simulink model "verify_Ventilation_AIV_mdl"  (R2016b)
settings: Solver=VariableStepDiscrete  StartTime=0  StopTime=1  MaxStep=1  RelTol=1e-3  EnableMultiTasking=on
undefined symbols (not defined in the file or in its folder): density, heat_capacity, rel_hum2x
libraries: carnot x3
settings Model: Creator=drhf  LastModifiedBy=drhf
settings DataIOCC: SaveFormat=Array  SignalLoggingSaveFormat=ModelDataLogs
settings OptimizationCC: ExpressionDepthLimit=2147483647  LifeSpan=inf
settings DebuggingCC: UnderspecifiedInitializationDetection=Classic  MergeDetectMultiDrivingBlocksExec=none  SolverPrmCheckMsg=warning  FcnCallInpInsideContextMsg=warning  StateNameClashWarn=warning  SFUnexpectedBacktrackingDiag=warning  SFNoUnconditionalDefaultTransitionDiag=warning  SFExecutionAtInitializationDiag=none
settings HardwareCC: ProdBitPerPointer=32  ProdBitPerSizeT=32  ProdBitPerPtrDiffT=32  ProdLargestAtomicFloat=None  ProdIntDivRoundTo=Undefined  ProdEndianess=Unspecified  ProdWordSize=32  ProdHWDeviceType=32-bit Generic
settings ModelReferenceCC: PropagateSignalLabelsOutOfModel=off
settings GRTTargetCC: TargetLangStandard=C89/C90 (ANSI)  GeneratePreprocessorConditionals=Disable all  CombineOutputUpdateFcns=off  GRTInterface=on
settings ConfigComp: CovMetricSettings=dw  CovHtmlReporting=on  CovSaveCumulativeToWorkspaceVar=on  CovSaveSingleToWorkspaceVar=on  CovExternalEMLEnable=off

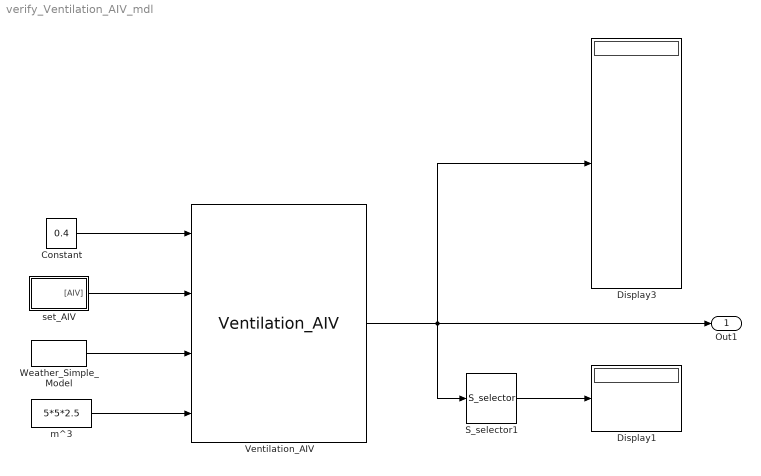
== system verify_Ventilation_AIV_mdl ==
  Constant : Constant  Value=0.4
  Display1 : Display
  Display3 : Display
  S_selector1 : carnot/Outputs/S_selector  e1=off  e2=off  e3=off  e4=off  e5=off  e6=off  e7=off  e8=off  e9=on  e10=on  e11=on  e12=off  e13=off
  Ventilation_AIV : carnot/Source/Ventilation/Ventilation_AIV  co2=400
  Weather_Simple_Model : carnot/Weather/Weather_Simple_Model  lat=60  Ibn=900  Idg=100  tamb=0  deltaTsky=0  rh=50  precip="10e-3/24/3600           % 10 mm in 24 h"  cloud=0.125  p=1013e2  vw=1  wdir=270
  m^3 : Constant  Value=5*5*2.5
  set_AIV : Subsystem
  Out1 : Outport
  wires:
  Constant/1 -> Ventilation_AIV/1
  set_AIV/1("[AIV]") -> Ventilation_AIV/2
  Weather_Simple_Model/1 -> Ventilation_AIV/3
  Ventilation_AIV/1 -> S_selector1/1, Display3/1, Out1/1
  m^3/1 -> Ventilation_AIV/4
  S_selector1/1 -> Display1/1

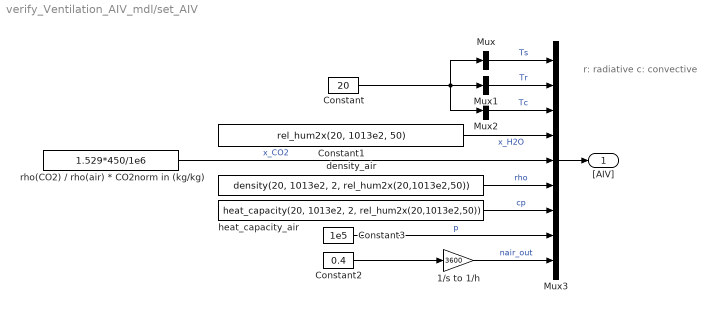
== system verify_Ventilation_AIV_mdl/set_AIV ==
  note: r: radiative
      | c: convective
  1/s to 1/h : Gain  Gain=3600  SaturateOnIntegerOverflow=on  OutDataTypeStr=Inherit: Same as input  ParamDataTypeStr=Inherit: Same as input
  Constant : Constant  Value=20
  Constant1 : Constant  Value=rel_hum2x(20, 1013e2, 50)
  Constant2 : Constant  Value=0.4
  Constant3 : Constant  Value=1e5
  Mux : Mux  Inputs=1
  Mux1 : Mux  Inputs=1
  Mux2 : Mux  Inputs=1
  Mux3 : Mux  Inputs=9
  density_air : Constant  Value=density(20, 1013e2, 2, rel_hum2x(20,1013e2,50))
  heat_capacity_air : Constant  Value=heat_capacity(20, 1013e2, 2, rel_hum2x(20,1013e2,50))
  rho(CO2) / rho(air) * CO2norm in (kg/kg) : Constant  Value=1.529*450/1e6
  "[AIV]" : Outport
  wires:
  Constant/1 -> Mux/1, Mux2/1, Mux1/1
  Mux3/1 -> "[AIV]"/1
  Constant2/1 -> 1/s to 1/h/1
  density_air/1 -> Mux3/6  "rho"
  heat_capacity_air/1 -> Mux3/7  "cp"
  Constant3/1 -> Mux3/8  "p"
  rho(CO2) / rho(air) * CO2norm in (kg/kg)/1 -> Mux3/5  "x_CO2"
  Constant1/1 -> Mux3/4  "x_H2O"
  1/s to 1/h/1 -> Mux3/9  "nair_out"
  Mux/1 -> Mux3/1  "Ts"
  Mux1/1 -> Mux3/2  "Tr"
  Mux2/1 -> Mux3/3  "Tc"
